simulink model "IMC_20140129"  (Simulink 7.9)
settings: Solver=ode14x  StartTime=0.0  StopTime=20  FixedStep=Ts  RelTol=1e-3
InitFcn:
  | IMC_ini
values from neighbouring files (symbols this model uses):
  Ts = 0.5    [IMC_calculo_limites_thetas.m]    (also in IMC_datta_ini.m; IMC_ini.m = 8.33333333333e-05; JORGE_controlador_LCL_malha_interna.m = 8.33333333333e-05; LCL_PAPM.m = 8.33333333333e-05)
undefined symbols (not defined in the file or in its folder): PD, PN
settings Model: Creator=Marcelo  LastModifiedBy=marcelodurgante
settings SolverCC: AutoInsertRateTranBlk=on
settings OptimizationCC: ExpressionDepthLimit=128
settings CodeAppCC: CustomSymbolStrType=$N$R$M_T
settings GRTTargetCC: CombineOutputUpdateFcns=off  GRTInterface=on

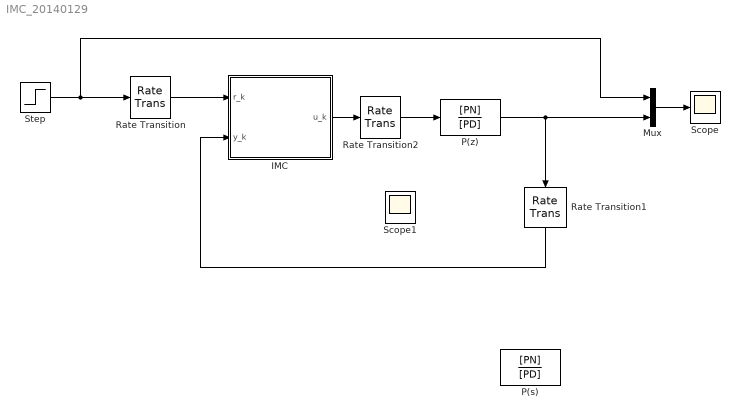
== system IMC_20140129 ==
  IMC : MATLAB Function  TreatAsAtomicUnit=on
  Mux : Mux  Inputs=2
  P(s) : TransferFcn  Numerator=[PN]  Denominator=[PD]
  P(z) : DiscreteTransferFcn  Numerator=[PN]  Denominator=[PD]  SampleTime=Ts
  Rate Transition : RateTransition  OutPortSampleTime=Ts
  Rate Transition1 : RateTransition  OutPortSampleTime=Ts
  Rate Transition2 : RateTransition  OutPortSampleTime=Ts
  Scope : Scope
  Scope1 : Scope
  Step : Step  Time=0.25  SampleTime=0
  wires:
  P(z)/1 -> Rate Transition1/1, Mux/2
  Mux/1 -> Scope/1
  Step/1 -> Rate Transition/1, Mux/1
  Rate Transition2/1 -> P(z)/1
  IMC/1(u_k) -> Rate Transition2/1
  Rate Transition/1 -> IMC/1(r_k)
  Rate Transition1/1 -> IMC/2(y_k)

== matlab function IMC ==
  data: r_k input double; y_k input double; u_k output double
function u_k = imc(r_k, y_k)
%#CODEGEN

%ganho adaptativo entre 0 e 0.5
gamma=0.1;

%constante escolhida entre 0 e 1
delta0=0.99;

%lambdas escolhidos de forma que Lambda seja estável
lambda0=0.0625;
lambda1=-0.5;
lambda2=1.5;
lambda3=-2;

%definição do conjunto no qual serão projetados os parâmetros
theta1_min=0.7046;
theta1_max=0.9532;
theta2_min=-1.5282;
theta2_max=-1.1296;
theta3_min= 0.425;
theta3_max= 0.575;
theta4_min= 0.0531;
theta4_max= 0.0719;
theta5_min= 5.0796e-04;
theta5_max= 6.8725e-04;
theta6_min= 0.002;
theta6_max= 0.0027;
theta7_min= 5.0796e-04;
theta7_max= 6.8725e-04;

%l é o grau do numerador e n é o grau do denominador da parte modelada da
%planta

%% Declarações

persistent theta_k;
if isempty(theta_k)
    theta_k=[0.8; -1.3; 0.5; 0.06; 6e-04; 0.0024; 6e-04];
end

persistent phi11_k1;
if isempty(phi11_k1)
    phi11_k1=0;
end

persistent phi11_k2;
if isempty(phi11_k2)
    phi11_k2=0;
end

persistent phi11_k3;
if isempty(phi11_k3)
    phi11_k3=0;
end

persistent phi11_k4;
if isempty(phi11_k4)
    phi11_k4=0;
end

persistent phi12_k1;
if isempty(phi12_k1)
    phi12_k1=0;
end

persistent phi12_k2;
if isempty(phi12_k2)
    phi12_k2=0;
end

persistent phi12_k3;
if isempty(phi12_k3)
    phi12_k3=0;
end

persistent phi12_k4;
if isempty(phi12_k4)
    phi12_k4=0;
end

persistent phi13_k1;
if isempty(phi13_k1)
    phi13_k1=0;
end

persistent phi13_k2;
if isempty(phi13_k2)
    phi13_k2=0;
end

persistent phi13_k3;
if isempty(phi13_k3)
    phi13_k3=0;
end

persistent phi13_k4;
if isempty(phi13_k4)
    phi13_k4=0;
end

persistent phi14_k1;
if isempty(phi14_k1)
    phi14_k1=0;
end

persistent phi14_k2;
if isempty(phi14_k2)
    phi14_k2=0;
end

persistent phi14_k3;
if isempty(phi14_k3)
    phi14_k3=0;
end

persistent phi14_k4;
if isempty(phi14_k4)
    phi14_k4=0;
end

persistent phi21_k1;
if isempty(phi21_k1)
    phi21_k1=0;
end

persistent phi21_k2;
if isempty(phi21_k2)
    phi21_k2=0;
end

persistent phi21_k3;
if isempty(phi21_k3)
    phi21_k3=0;
end

persistent phi21_k4;
if isempty(phi21_k4)
    phi21_k4=0;
end

persistent phi22_k1;
if isempty(phi22_k1)
    phi22_k1=0;
end

persistent phi22_k2;
if isempty(phi22_k2)
    phi22_k2=0;
end

persistent phi22_k3;
if isempty(phi22_k3)
    phi22_k3=0;
end

persistent phi22_k4;
if isempty(phi22_k4)
    phi22_k4=0;
end

persistent phi23_k1;
if isempty(phi23_k1)
    phi23_k1=0;
end

persistent phi23_k2;
if isempty(phi23_k2)
    phi23_k2=0;
end

persistent phi23_k3;
if isempty(phi23_k3)
    phi23_k3=0;
end

persistent phi23_k4;
if isempty(phi23_k4)
    phi23_k4=0;
end

persistent u_k1;
if isempty(u_k1)
    u_k1=0;
end

persistent u_k2;
if isempty(u_k2)
    u_k2=0;
end

persistent u_k3;
if isempty(u_k3)
    u_k3=0;
end

persistent u_k4;
if isempty(u_k4)
    u_k4=0;
end

persistent y_k1;
if isempty(y_k1)
    y_k1=0;
end

persistent y_k2;
if isempty(y_k2)
    y_k2=0;
end

persistent y_k3;
if isempty(y_k3)
    y_k3=0;
end

persistent y_k4;
if isempty(y_k4)
    y_k4=0;
end

persistent rer_k1;
if isempty(rer_k1)
    rer_k1=0;
end

persistent rer_k2;
if isempty(rer_k2)
    rer_k2=0;
end

persistent rer_k3;
if isempty(rer_k3)
    rer_k3=0;
end

persistent rer_k4;
if isempty(rer_k4)
    rer_k4=0;
end

persistent m2;
if isempty(m2)
    m2=1;
end

persistent count;
if isempty(count)
    count=0;
end

%% Cálculos

phi11_k = y_k1 - lambda3*phi11_k1 - lambda2*phi11_k2 - lambda1*phi11_k3 - lambda0*phi11_k4;
phi12_k = y_k2 - lambda3*phi12_k1 - lambda2*phi12_k2 - lambda1*phi12_k3 - lambda0*phi12_k4;
phi13_k = y_k3 - lambda3*phi13_k1 - lambda2*phi13_k2 - lambda1*phi13_k3 - lambda0*phi13_k4;
phi14_k = y_k4 - lambda3*phi14_k1 - lambda2*phi14_k2 - lambda1*phi14_k3 - lambda0*phi14_k4;
phi21_k = u_k2 - lambda3*phi21_k1 - lambda2*phi21_k2 - lambda1*phi21_k3 - lambda0*phi21_k4;
phi22_k = u_k3 - lambda3*phi22_k1 - lambda2*phi22_k2 - lambda1*phi22_k3 - lambda0*phi22_k4;
phi23_k = u_k4 - lambda3*phi23_k1 - lambda2*phi23_k2 - lambda1*phi23_k3 - lambda0*phi23_k4;

phi1_k=[phi11_k phi12_k phi13_k phi14_k];
phi2_k=[phi21_k phi22_k phi23_k];

phi_k = [phi1_k'; phi2_k'];

m2_k= m2 + phi_k'*phi_k;

y_hat_k= theta_k'*phi_k;

eta_k= (y_k - y_hat_k)/m2_k;

%calculo da acao de controle
%delta_b=real(sqrt(complex(theta_k(6)^2-4*theta_k(5)*theta_k(7))));
delta_b=theta_k(6)^2-4*theta_k(5)*theta_k(7);
phi=2*theta_k(5)/(-theta_k(6)-delta_b);
rer_k= r_k - (y_k - y_hat_k);
ganho_controlador=(1-phi)/(1-(1/phi));
%ganho_controlador=1;
z_fm=(-theta_k(6)+delta_b)/(2*theta_k(5));
%z_nm=(-theta_k(6)-delta_b)/(2*theta_k(5));
u_k= ganho_controlador*(rer_k + (lambda3-theta_k(1))*rer_k1 + (lambda2-theta_k(2))*rer_k2 + (lambda1-theta_k(3))*rer_k3 + (lambda0-theta_k(4))*rer_k4) ...
    - ((2*(theta_k(5)-theta_k(7)))/(theta_k(6)+delta_b))*u_k1 - ((theta_k(6)-delta_b)/(theta_k(6)+delta_b))*u_k2;


%% Atualização

m2 = delta0*(m2 - 1) + u_k^2 + y_k^2 + 1;

%atualização de theta_k via algoritmo de projeção de parâmetros
g1_k= -gamma*eta_k*phi11_k;
g2_k= -gamma*eta_k*phi12_k;
g3_k= -gamma*eta_k*phi13_k;
g4_k= -gamma*eta_k*phi14_k;
g5_k= -gamma*eta_k*phi21_k;
g6_k= -gamma*eta_k*phi22_k;
g7_k= -gamma*eta_k*phi23_k;

f1_k=0;
if (theta_k(1)+g1_k)>theta1_max
    f1_k=theta1_max-theta_k(1)-g1_k;
end
if (theta_k(1)+g1_k)<theta1_min
    f1_k=theta1_min-theta_k(1)-g1_k;
end

f2_k=0;
if (theta_k(2)+g2_k)>theta2_max
    f2_k=theta2_max-theta_k(2)-g2_k;
end
if (theta_k(2)+g2_k)<theta2_min
    f2_k=theta2_min-theta_k(2)-g2_k;
end

f3_k=0;
if (theta_k(3)+g3_k)>theta3_max
    f3_k=theta3_max-theta_k(3)-g3_k;
end
if (theta_k(3)+g3_k)<theta3_min
    f3_k=theta3_min-theta_k(3)-g3_k;
end

f4_k=0;
if (theta_k(4)+g4_k)>theta4_max
    f4_k=theta4_max-theta_k(4)-g4_k;
end
if (theta_k(4)+g4_k)<theta4_min
    f4_k=theta4_min-theta_k(4)-g4_k;
end

f5_k=0;
if (theta_k(5)+g5_k)>theta5_max
    f5_k=theta5_max-theta_k(5)-g5_k;
end
if (theta_k(5)+g5_k)<theta5_min
    f5_k=theta5_min-theta_k(5)-g5_k;
end

f6_k=0;
if (theta_k(6)+g6_k)>theta6_max
    f6_k=theta6_max-theta_k(6)-g6_k;
end
if (theta_k(6)+g6_k)<theta6_min
    f6_k=theta6_min-theta_k(6)-g6_k;
end

f7_k=0;
if (theta_k(7)+g7_k)>theta7_max
    f7_k=theta7_max-theta_k(7)-g7_k;
end
if (theta_k(7)+g7_k)<theta7_min
    f7_k=theta7_min-theta_k(7)-g7_k;
end

f_k = [f1_k; f2_k; f3_k; f4_k; f5_k; f6_k; f7_k];

%theta_k = theta_k + gamma*eta_k*phi_k + f_k;

thetas = theta_k;


%atualização de estados anteriores
phi11_k4 = phi11_k3;
phi11_k3 = phi11_k2;
phi11_k2 = phi11_k1;
phi11_k1 = phi11_k;
phi12_k4 = phi12_k3;
phi12_k3 = phi12_k2;
phi12_k2 = phi12_k1;
phi12_k1 = phi12_k;
phi13_k4 = phi13_k3;
phi13_k3 = phi13_k2;
phi13_k2 = phi13_k1;
phi13_k1 = phi13_k;
phi14_k4 = phi14_k3;
phi14_k3 = phi14_k2;
phi14_k2 = phi14_k1;
phi14_k1 = phi14_k;
phi21_k4 = phi21_k3;
phi21_k3 = phi21_k2;
phi21_k2 = phi21_k1;
phi21_k1 = phi21_k;
phi22_k4 = phi22_k3;
phi22_k3 = phi22_k2;
phi22_k2 = phi22_k1;
phi22_k1 = phi22_k;
phi23_k4 = phi23_k3;
phi23_k3 = phi23_k2;
phi23_k2 = phi23_k1;
phi23_k1 = phi23_k;

u_k4 = u_k3;
u_k3 = u_k2;
u_k2 = u_k1;
u_k1 = u_k;

y_k4 = y_k3;
y_k3 = y_k2;
y_k2 = y_k1;
y_k1 = y_k;

rer_k4 = rer_k3;
rer_k3 = rer_k2;
rer_k2 = rer_k1;
rer_k1 = rer_k;


end
